simulink model "Fig524"  (R2014b)
settings: Solver=ode3  StartTime=0.0  StopTime=0.1048576  FixedStep=2e-7  RelTol=1e-3
libraries: commseqgen2 x1, commutil2 x1, commanapbnd3 x1, commrandsrc2 x1, powerlib_meascontrol x1
settings Model: Creator=Silage  LastModifiedBy=Silage

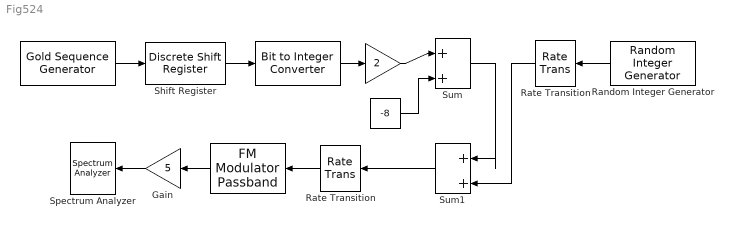
== system Fig524 ==
  " " : commseqgen2/Gold Sequence Generator  genPoly1=[1 0 0 1 0 1]  iniState1=[1 1 1 0 1]  genPoly2=[1 1 1 1 0 1]  iniState2=[1 0 0 0 1]  index=0  shift=0  outVarSiz=off  maxOutSizeMode=Dialog parameter  maxOutSize=[10 1]  ts=5e-5  frameBased=off  sampPerFrame=1  reset=off  outDataType=double
  "  " : commutil2/Bit to Integer Converter  nbits=3  bitOrder=MSB first  signedOutputValues=Unsigned  outDtype=Inherit via internal rule  outDtypeSigned=Inherit via internal rule
  "   " : Gain  Gain=2
  "    " : Constant  Value=-8
  "        " : commanapbnd3/FM Modulator Passband  Fc=100000  Ph=0  Kc=5000
  Gain : Gain  Gain=5
  Random Integer Generator : commrandsrc2/Random Integer Generator  mul=2  seed=randseed  Ts=1e-3  frameBased=off  sampPerFrame=50  orient=on  outDataType=double
  Rate Transition : RateTransition  OutPortSampleTime=2e-7
  Rate Transition : RateTransition  OutPortSampleTime=5e-5
  Shift Register : powerlib_meascontrol/Additional Components/Discrete Shift Register  NSamples=3  InitialValue=0  Ts=5e-5
  Spectrum Analyzer : SpectrumAnalyzer
  Sum : Sum  Inputs=|++
  Sum1 : Sum  Inputs=|++
  wires:
  Random Integer Generator/1 -> Rate Transition/1
  Gain/1 -> Spectrum Analyzer/1
  "        "/1 -> Gain/1
  " "/1 -> Shift Register/1
  Shift Register/1 -> "  "/1
  "  "/1 -> "   "/1
  Sum1/1 -> Rate Transition/1
  Rate Transition/1 -> "        "/1
  Sum/1 -> Sum1/1
  Rate Transition/1 -> Sum1/2
  "    "/1 -> Sum/2
  "   "/1 -> Sum/1
